simulink model "Observer_Controller"  (R2022a)
settings: Solver=ode45  StartTime=0.0  StopTime=20  RelTol=1e-3
values from neighbouring files (symbols this model uses):
  A = [0 0 1 0 0 ... (first row only)    [DesignProjectP2.m]    (also in DesignProjectP3.m; DesignProject_OffsetP3.m; mpc_example_regulation.m = [ 	 0,       0,              1,  0, 0; 	 0,       0,        ; mpc_example_tracking.m = [ 	 0,       0,              1,  0, 0; 	 0,       0,        )
  A_11 = A_measured(:,1:2)    [DesignProjectP2.m]
  A_12 = A_measured(:,3:5)    [DesignProjectP2.m]
  A_21 = A_estimated(:,1:2)    [DesignProjectP2.m]
  A_22 = A_estimated(:,3:5)    [DesignProjectP2.m]
  absolute_encoder_counts_per_revolution = 4096    [ELEN90064_Project_Parameters.m]
  B = [0;0;0;0;1/La]    [DesignProjectP2.m]    (also in DesignProjectP3.m; DesignProject_OffsetP3.m; mpc_example_regulation.m = [0; 0; 0; 0; 1/La]; mpc_example_tracking.m = [0; 0; 0; 0; 1/La])
  B_1 = [Dp.b(1); Dp.b(2)]    [DesignProjectP2.m]
  B_2 = [Dp.b(3); Dp.b(4); Dp.b(5)]    [DesignProjectP2.m]
  C = [1 0 0 0 0 ... (first row only)    [DesignProjectP2.m]    (also in DesignProjectP3.m; DesignProject_OffsetP3.m; mpc_example_regulation.m; mpc_example_tracking.m)
  init = [theta_m_init; theta_l_init; thetadot_m_init; thetadot_l_init; Ia_init]    [ELEN90064_Project_Parameters.m]
  J_r = place(A_22', A_12', obsz)'    [DesignProjectP2.m]
  K = K(2:6)    [DesignProjectP2.m]    (also in DesignProjectP3.m; DesignProject_OffsetP3.m = K_dist(2:6); phase2_emc.m = place(A,B,desired_poles))
  K_disc = K_disc(2:6)    [DesignProjectP2.m]    (also in DesignProject_OffsetP3.m = Kr_disc(2:6))
  Ki = K(1)    [DesignProjectP2.m]    (also in DesignProjectP3.m; DesignProject_OffsetP3.m = K_dist(1))
  Ki_disc = K_disc(1)    [DesignProjectP2.m]    (also in DesignProject_OffsetP3.m = Kr_disc(1))
  L = place(A', C', observer_poles)'    [DesignProjectP2.m]    (also in DesignProjectP3.m; DesignProject_OffsetP3.m = L_t'; phase2_emc.m = place(A',C',desired_obsv_poles)')
  theta_l_init = deg2rad(0)    [ELEN90064_Project_Parameters.m]    (also in mpc_example_regulation.m; mpc_example_tracking.m)
  vision_fps = 50    [ELEN90064_Project_Parameters.m]
settings Model: Creator=Admin  LastModifiedBy=Admin

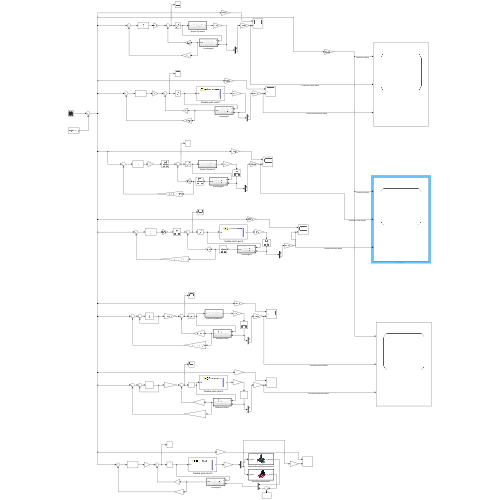
[thumbnail: Simulink's stored preview of the top-level diagram]
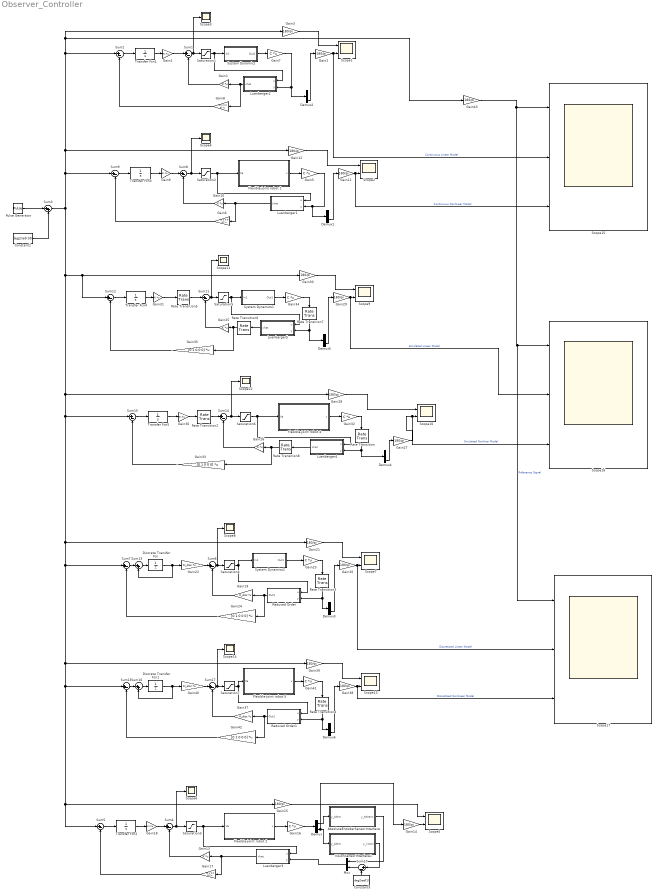
== system Observer_Controller ==
  AbsoluteEncoderSensorInterface : Subsystem  TreatAsAtomicUnit=on
      mask Display: image('$imagefile'); % Use "Edit Image" on toolstrip to change.
  Constant1 : Constant  Value=deg2rad(30)
  Constant3 : Constant  Value=deg2rad(1)
  Demux{,1..6} (7 alike) : Demux  Outputs=2
  Discrete Transfer Fcn : DiscreteTransferFcn  Denominator=[1 0]
  Discrete Transfer Fcn1 : DiscreteTransferFcn  Denominator=[1 0]
  Flexible-joint robot 1 : Subsystem
      mask Display: image('$imagefile'); % Use "Edit Image" on toolstrip to change.
  Flexible-joint robot 2 : Subsystem
      mask Display: image('$imagefile'); % Use "Edit Image" on toolstrip to change.
  Flexible-joint robot 4 : Subsystem
      mask Display: image('$imagefile'); % Use "Edit Image" on toolstrip to change.
  Flexible-joint robot 5 : Subsystem
      mask Display: image('$imagefile'); % Use "Edit Image" on toolstrip to change.
  Gain{1,10,13,25..26} (5 alike) : Gain  Gain=K  Multiplication=Matrix(K*u)
  Gain{2..3,11..12,14..15,20..21,27..30,38..39,43} (15 alike) : Gain  Gain=180/pi
  Gain{5,7,16,23,32,34,41} (7 alike) : Gain  Gain=C  Multiplication=Matrix(K*u)
  Gain{6,8,17,24,33,35,42} (7 alike) : Gain  Gain=[0 1 0 0 0]  Multiplication=Matrix(K*u)
  Gain{4,9,18,31,36} (5 alike) : Gain  Gain=Ki  Multiplication=Matrix(K*u)
  Gain19 : Gain  Gain=K_disc  Multiplication=Matrix(K*u)
  Gain22 : Gain  Gain=Ki_disc  Multiplication=Matrix(K*u)
  Gain37 : Gain  Gain=K_disc  Multiplication=Matrix(K*u)
  Gain40 : Gain  Gain=Ki_disc  Multiplication=Matrix(K*u)
  Luenberger1 : Subsystem  TreatAsAtomicUnit=on
  Luenberger2 : Subsystem  TreatAsAtomicUnit=on
  Luenberger3 : Subsystem  TreatAsAtomicUnit=on
  Luenberger4 : Subsystem  TreatAsAtomicUnit=on
  Luenberger5 : Subsystem  TreatAsAtomicUnit=on
  Mux : Mux  Inputs=2
  Pulse Generator : DiscretePulseGenerator  PulseType=Time based  Amplitude=deg2rad(30)  Period=5  PulseWidth=50
  Rate Transition{,2..8} (8 alike) : RateTransition  OutPortSampleTime=T
  Reduced Order : Subsystem  TreatAsAtomicUnit=on
  Reduced Order1 : Subsystem  TreatAsAtomicUnit=on
  Saturation{1..7} (7 alike) : Saturate  UpperLimit=6  LowerLimit=-6
  Scope{1..2,5,7,9..10,13} (7 alike) : Scope  NumInputPorts=2
  Scope{3..4,6,8,11..12,14} (7 alike) : Scope
  Scope15 : Scope  NumInputPorts=3
  Scope16 : Scope  NumInputPorts=3
  Scope17 : Scope  NumInputPorts=3
  Sum{1..2,4..12,14..15,17..18} (15 alike) : Sum  Inputs=|+-
  Sum13 : Sum  Inputs=|++
  Sum16 : Sum  Inputs=|++
  Sum3 : Sum  Inputs=|++
  System Dynamics : Subsystem  TreatAsAtomicUnit=on
  System Dynamics1 : Subsystem  TreatAsAtomicUnit=on
  System Dynamics2 : Subsystem  TreatAsAtomicUnit=on
  Transfer Fcn{1..5} (5 alike) : TransferFcn  Denominator=[1 0]
  VisionSensorInterface1 : Subsystem  TreatAsAtomicUnit=on
      mask Display: image('$imagefile'); % Use "Edit Image" on toolstrip to change.
  wires:
  Sum8/1 -> Scope4/1, Saturation2/1
  Saturation2/1 -> Luenberger1/1(u), Flexible-joint robot 1/1(Va)
  Sum9/1 -> Transfer Fcn3/1
  Gain10/1 -> Sum8/2
  Transfer Fcn3/1 -> Gain9/1
  Flexible-joint robot 1/1(x) -> Gain5/1
  Gain12/1 -> Scope2/1
  Gain11/1 -> Scope15/3, Scope2/2  "Continuous Nonlinear Model"
  Gain5/1 -> Demux1/1, Luenberger1/2(y)
  Luenberger1/1(xhat) -> Gain6/1, Gain10/1
  Gain6/1 -> Sum9/2
  Gain9/1 -> Sum8/1
  Gain2/1 -> Scope15/2, Scope1/2  "Continuous Linear Model"
  Gain3/1 -> Scope1/1
  Transfer Fcn1/1 -> Gain4/1
  Gain1/1 -> Sum1/2
  Sum2/1 -> Transfer Fcn1/1
  Sum1/1 -> Scope3/1, Saturation1/1
  Gain8/1 -> Sum2/2
  Gain4/1 -> Sum1/1
  Saturation1/1 -> Luenberger2/1(u), System Dynamics/1(In1)
  Luenberger2/1(xhat) -> Gain8/1, Gain1/1
  Pulse Generator/1 -> Sum3/1
  System Dynamics/1(Out1) -> Gain7/1
  Luenberger3/1(xhat) -> Gain17/1, Gain13/1
  Saturation3/1 -> Luenberger3/1(u), Flexible-joint robot 2/1(Va)
  Flexible-joint robot 2/1(x) -> Gain16/1
  Gain13/1 -> Sum4/2
  Gain14/1 -> Scope5/2
  Gain18/1 -> Sum4/1
  Sum5/1 -> Transfer Fcn2/1
  Sum4/1 -> Scope6/1, Saturation3/1
  Transfer Fcn2/1 -> Gain18/1
  Gain17/1 -> Sum5/2
  Gain15/1 -> Scope5/1
  Constant1/1 -> Sum3/2
  Gain16/1 -> Demux/1
  Demux/1 -> AbsoluteEncoderSensorInterface/1(y_plant)
  AbsoluteEncoderSensorInterface/1(y_absenc) -> Mux/1
  Demux/2 -> Gain14/1, VisionSensorInterface1/1(y_plant)
  Mux/1 -> Luenberger3/2(y)
  System Dynamics2/1(Out1) -> Gain23/1
  Reduced Order/1(Out1) -> Gain24/1, Gain19/1
  Saturation4/1 -> System Dynamics2/1(In1), Reduced Order/1(u)
  Gain22/1 -> Sum6/1
  Gain24/1 -> Sum7/2
  Sum6/1 -> Saturation4/1, Scope8/1
  Gain19/1 -> Sum6/2
  Gain21/1 -> Scope7/1
  Gain20/1 -> Scope17/2, Scope7/2  "Discretised Linear Model"
  VisionSensorInterface1/1(y_vision) -> Sum10/1
  Constant3/1 -> Sum10/2
  Sum10/1 -> Mux/2
  Demux1/2 -> Gain11/1
  Sum13/1 -> Discrete Transfer Fcn/1
  Discrete Transfer Fcn/1 -> Gain22/1, Sum13/2
  Sum7/1 -> Sum13/1
  Demux2/2 -> Gain2/1
  Gain7/1 -> Demux2/1, Luenberger2/2(y)
  Gain23/1 -> Rate Transition3/1
  Demux3/2 -> Gain20/1
  Gain34/1 -> Rate Transition7/1
  Demux5/2 -> Gain29/1
  Demux4/2 -> Gain27/1
  System Dynamics1/1(Out1) -> Gain34/1
  Luenberger5/1(xhat) -> Rate Transition6/1
  Saturation5/1 -> System Dynamics1/1(In1), Luenberger5/1(u)
  Gain31/1 -> Rate Transition5/1
  Gain35/1 -> Sum12/2
  Sum11/1 -> Saturation5/1, Scope11/1
  Sum12/1 -> Transfer Fcn4/1
  Gain25/1 -> Sum11/2
  Transfer Fcn4/1 -> Gain31/1
  Gain30/1 -> Scope9/1
  Gain29/1 -> Scope16/2, Scope9/2  "Emulated Linear Model"
  Gain36/1 -> Rate Transition2/1
  Gain33/1 -> Sum15/2
  Luenberger4/1(xhat) -> Rate Transition8/1
  Gain32/1 -> Rate Transition/1
  Gain27/1 -> Scope16/3, Scope10/2  "Emulated Nonliner Model"
  Gain28/1 -> Scope10/1
  Flexible-joint robot 4/1(x) -> Gain32/1
  Transfer Fcn5/1 -> Gain36/1
  Sum15/1 -> Transfer Fcn5/1
  Saturation6/1 -> Flexible-joint robot 4/1(Va), Luenberger4/1(u)
  Sum14/1 -> Saturation6/1, Scope12/1
  Rate Transition/1 -> Demux4/1, Luenberger4/2(y)
  Gain26/1 -> Sum14/2
  Rate Transition2/1 -> Sum14/1
  Sum3/1 -> Gain12/1, Gain3/1, Gain43/1, Sum2/1, Sum9/1, Sum12/1, Gain30/1, Gain28/1, Gain21/1, Gain39/1, Sum5/1, Gain15/1, Sum18/1, Sum7/1, Sum15/1
  Demux6/2 -> Gain38/1
  Gain41/1 -> Rate Transition4/1
  Sum18/1 -> Sum16/1
  Discrete Transfer Fcn1/1 -> Sum16/2, Gain40/1
  Sum16/1 -> Discrete Transfer Fcn1/1
  Gain38/1 -> Scope17/3, Scope13/2  "Discretised Nonlinear Model"
  Gain39/1 -> Scope13/1
  Gain37/1 -> Sum17/2
  Sum17/1 -> Scope14/1, Saturation7/1
  Gain42/1 -> Sum18/2
  Gain40/1 -> Sum17/1
  Saturation7/1 -> Reduced Order1/1(u), Flexible-joint robot 5/1(Va)
  Reduced Order1/1(Out1) -> Gain37/1, Gain42/1
  Flexible-joint robot 5/1(x) -> Gain41/1
  Rate Transition3/1 -> Demux3/1, Reduced Order/2(y)
  Rate Transition4/1 -> Demux6/1, Reduced Order1/2(y)
  Rate Transition5/1 -> Sum11/1
  Rate Transition6/1 -> Gain35/1, Gain25/1
  Rate Transition7/1 -> Luenberger5/2(y), Demux5/1
  Gain43/1 -> Scope17/1, Scope16/1, Scope15/1  "Reference Signal"
  Rate Transition8/1 -> Gain33/1, Gain26/1

== system Observer_Controller/AbsoluteEncoderSensorInterface ==
  note: Notes:
      | > This sensor block is protected.
      | > The AbsoluteEncoderSensor.slxp file needs to be on the Matlab path in order to simulate this sensor.
      | > You should have download the .slpx file appropriate for you operating system {Windows, Mac, Linux}.
      | > The constant parameters on the left are set in the " ELEN90064_Project_Parameters.m " script.
      | > The sensors appendix in project description provides a 1-page summary of the sensor model and of how each parameters relates to the expected performance of the sensor.
      | > You should read the relevant page of that appendix before using this sensor.
  y_plant : Inport
  AbsoluteEncoderSensor : ModelReference  ModelNameDialog=AbsoluteEncoderSensor.slxp  ModelReferenceVersion=1.16  CopyOfModelProtected=on
  NUMBER OF COUNTS PER REVOLUTION : Constant  Value=absolute_encoder_counts_per_revolution
  y_absenc : Outport
  wires:
  NUMBER OF COUNTS PER REVOLUTION/1 -> AbsoluteEncoderSensor/1
  y_plant/1 -> AbsoluteEncoderSensor/2
  AbsoluteEncoderSensor/1 -> y_absenc/1

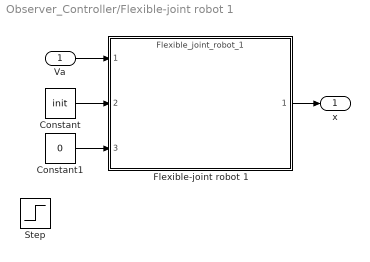
== system Observer_Controller/Flexible-joint robot 1 ==
  Va : Inport
  Constant : Constant  Value=init
  Constant1 : Constant  Value=0
  Flexible-joint robot 1 : ModelReference  ModelNameDialog=Flexible_joint_robot_1  ModelReferenceVersion=1.65  CopyOfModelProtected=on
  Step : Step  After=0.05  SampleTime=0
  x : Outport
  wires:
  Constant/1 -> Flexible-joint robot 1/2
  Constant1/1 -> Flexible-joint robot 1/3
  Flexible-joint robot 1/1 -> x/1
  Va/1 -> Flexible-joint robot 1/1

== system Observer_Controller/Flexible-joint robot 2 ==
  Va : Inport
  Constant : Constant  Value=init
  Constant1 : Constant  Value=0
  Flexible-joint robot 1 : ModelReference  ModelNameDialog=Flexible_joint_robot_1  ModelReferenceVersion=1.65  CopyOfModelProtected=on
  x : Outport
  wires:
  Constant/1 -> Flexible-joint robot 1/2
  Constant1/1 -> Flexible-joint robot 1/3
  Flexible-joint robot 1/1 -> x/1
  Va/1 -> Flexible-joint robot 1/1

== system Observer_Controller/Flexible-joint robot 4 ==
  Va : Inport
  Constant : Constant  Value=init
  Constant1 : Constant  Value=0
  Flexible-joint robot 1 : ModelReference  ModelNameDialog=Flexible_joint_robot_1  ModelReferenceVersion=1.65  CopyOfModelProtected=on
  Step : Step  After=0.05  SampleTime=0
  x : Outport
  wires:
  Va/1 -> Flexible-joint robot 1/1
  Flexible-joint robot 1/1 -> x/1
  Constant1/1 -> Flexible-joint robot 1/3
  Constant/1 -> Flexible-joint robot 1/2

== system Observer_Controller/Flexible-joint robot 5 ==
  Va : Inport
  Constant : Constant  Value=init
  Constant1 : Constant  Value=0
  Flexible-joint robot 1 : ModelReference  ModelNameDialog=Flexible_joint_robot_1  ModelReferenceVersion=1.65  CopyOfModelProtected=on
  Step : Step  After=0.05  SampleTime=0
  x : Outport
  wires:
  Constant/1 -> Flexible-joint robot 1/2
  Constant1/1 -> Flexible-joint robot 1/3
  Flexible-joint robot 1/1 -> x/1
  Va/1 -> Flexible-joint robot 1/1

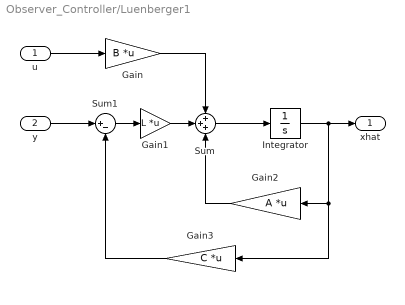
== system Observer_Controller/Luenberger1 ==
  u : Inport
  y : Inport  Port=2
  Gain : Gain  Gain=B  Multiplication=Matrix(K*u) (u vector)
  Gain1 : Gain  Gain=L  Multiplication=Matrix(K*u) (u vector)
  Gain2 : Gain  Gain=A  Multiplication=Matrix(K*u) (u vector)
  Gain3 : Gain  Gain=C  Multiplication=Matrix(K*u) (u vector)
  Integrator : Integrator
  Sum : Sum  Inputs=+++
  Sum1 : Sum  Inputs=|+-
  xhat : Outport
  wires:
  u/1 -> Gain/1
  Gain/1 -> Sum/1
  y/1 -> Sum1/1
  Sum1/1 -> Gain1/1
  Gain1/1 -> Sum/2
  Sum/1 -> Integrator/1
  Integrator/1 -> Gain3/1, Gain2/1, xhat/1
  Gain2/1 -> Sum/3
  Gain3/1 -> Sum1/2

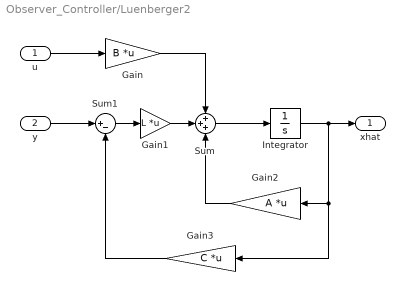
== system Observer_Controller/Luenberger2 ==
  u : Inport
  y : Inport  Port=2
  Gain : Gain  Gain=B  Multiplication=Matrix(K*u) (u vector)
  Gain1 : Gain  Gain=L  Multiplication=Matrix(K*u) (u vector)
  Gain2 : Gain  Gain=A  Multiplication=Matrix(K*u) (u vector)
  Gain3 : Gain  Gain=C  Multiplication=Matrix(K*u) (u vector)
  Integrator : Integrator
  Sum : Sum  Inputs=+++
  Sum1 : Sum  Inputs=|+-
  xhat : Outport
  wires:
  u/1 -> Gain/1
  Gain/1 -> Sum/1
  y/1 -> Sum1/1
  Sum1/1 -> Gain1/1
  Gain1/1 -> Sum/2
  Sum/1 -> Integrator/1
  Integrator/1 -> Gain3/1, Gain2/1, xhat/1
  Gain2/1 -> Sum/3
  Gain3/1 -> Sum1/2

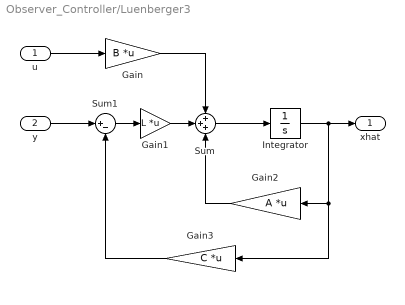
== system Observer_Controller/Luenberger3 ==
  u : Inport
  y : Inport  Port=2
  Gain : Gain  Gain=B  Multiplication=Matrix(K*u) (u vector)
  Gain1 : Gain  Gain=L  Multiplication=Matrix(K*u) (u vector)
  Gain2 : Gain  Gain=A  Multiplication=Matrix(K*u) (u vector)
  Gain3 : Gain  Gain=C  Multiplication=Matrix(K*u) (u vector)
  Integrator : Integrator
  Sum : Sum  Inputs=+++
  Sum1 : Sum  Inputs=|+-
  xhat : Outport
  wires:
  u/1 -> Gain/1
  Gain/1 -> Sum/1
  y/1 -> Sum1/1
  Sum1/1 -> Gain1/1
  Gain1/1 -> Sum/2
  Sum/1 -> Integrator/1
  Integrator/1 -> Gain3/1, Gain2/1, xhat/1
  Gain2/1 -> Sum/3
  Gain3/1 -> Sum1/2

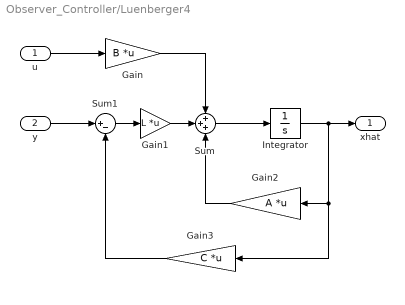
== system Observer_Controller/Luenberger4 ==
  u : Inport
  y : Inport  Port=2
  Gain : Gain  Gain=B  Multiplication=Matrix(K*u) (u vector)
  Gain1 : Gain  Gain=L  Multiplication=Matrix(K*u) (u vector)
  Gain2 : Gain  Gain=A  Multiplication=Matrix(K*u) (u vector)
  Gain3 : Gain  Gain=C  Multiplication=Matrix(K*u) (u vector)
  Integrator : Integrator
  Sum : Sum  Inputs=+++
  Sum1 : Sum  Inputs=|+-
  xhat : Outport
  wires:
  Gain3/1 -> Sum1/2
  Gain2/1 -> Sum/3
  Integrator/1 -> xhat/1, Gain2/1, Gain3/1
  Sum/1 -> Integrator/1
  Gain1/1 -> Sum/2
  Sum1/1 -> Gain1/1
  y/1 -> Sum1/1
  Gain/1 -> Sum/1
  u/1 -> Gain/1

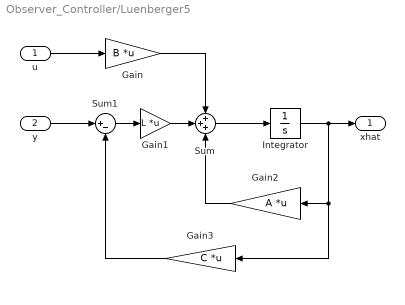
== system Observer_Controller/Luenberger5 ==
  u : Inport
  y : Inport  Port=2
  Gain : Gain  Gain=B  Multiplication=Matrix(K*u) (u vector)
  Gain1 : Gain  Gain=L  Multiplication=Matrix(K*u) (u vector)
  Gain2 : Gain  Gain=A  Multiplication=Matrix(K*u) (u vector)
  Gain3 : Gain  Gain=C  Multiplication=Matrix(K*u) (u vector)
  Integrator : Integrator
  Sum : Sum  Inputs=+++
  Sum1 : Sum  Inputs=|+-
  xhat : Outport
  wires:
  Gain3/1 -> Sum1/2
  Gain2/1 -> Sum/3
  Integrator/1 -> xhat/1, Gain2/1, Gain3/1
  Sum/1 -> Integrator/1
  Gain1/1 -> Sum/2
  Sum1/1 -> Gain1/1
  y/1 -> Sum1/1
  Gain/1 -> Sum/1
  u/1 -> Gain/1

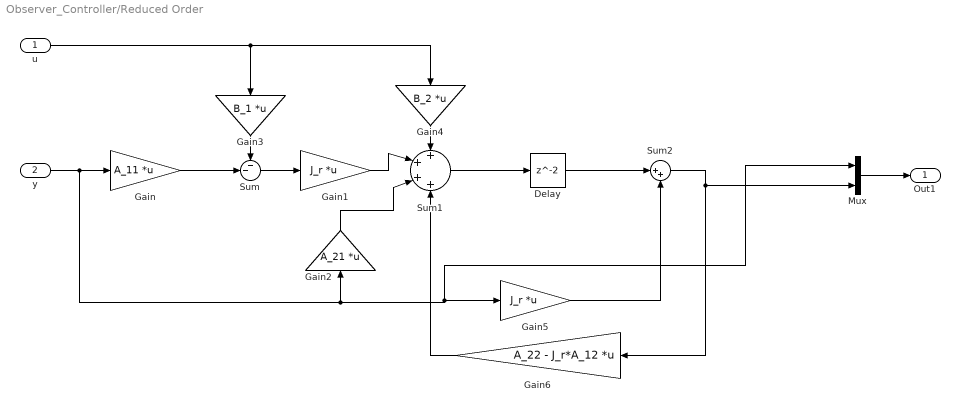
== system Observer_Controller/Reduced Order ==
  u : Inport
  y : Inport  Port=2
  Delay : Delay
  Gain : Gain  Gain=A_11  Multiplication=Matrix(K*u) (u vector)
  Gain1 : Gain  Gain=J_r  Multiplication=Matrix(K*u) (u vector)
  Gain2 : Gain  Gain=A_21  Multiplication=Matrix(K*u) (u vector)
  Gain3 : Gain  Gain=B_1  Multiplication=Matrix(K*u) (u vector)
  Gain4 : Gain  Gain=B_2  Multiplication=Matrix(K*u) (u vector)
  Gain5 : Gain  Gain=J_r  Multiplication=Matrix(K*u) (u vector)
  Gain6 : Gain  Gain=A_22 - J_r*A_12  Multiplication=Matrix(K*u) (u vector)
  Mux : Mux  Inputs=2
  Sum : Sum  Inputs=--|
  Sum1 : Sum  Inputs=++++
  Sum2 : Sum  Inputs=|++
  Out1 : Outport
  wires:
  u/1 -> Gain4/1, Gain3/1
  y/1 -> Gain2/1, Mux/1, Gain5/1, Gain/1
  Gain/1 -> Sum/2
  Sum/1 -> Gain1/1
  Gain1/1 -> Sum1/2
  Gain2/1 -> Sum1/3
  Gain3/1 -> Sum/1
  Gain4/1 -> Sum1/1
  Sum1/1 -> Delay/1
  Gain5/1 -> Sum2/2
  Delay/1 -> Sum2/1
  Gain6/1 -> Sum1/4
  Sum2/1 -> Gain6/1, Mux/2
  Mux/1 -> Out1/1

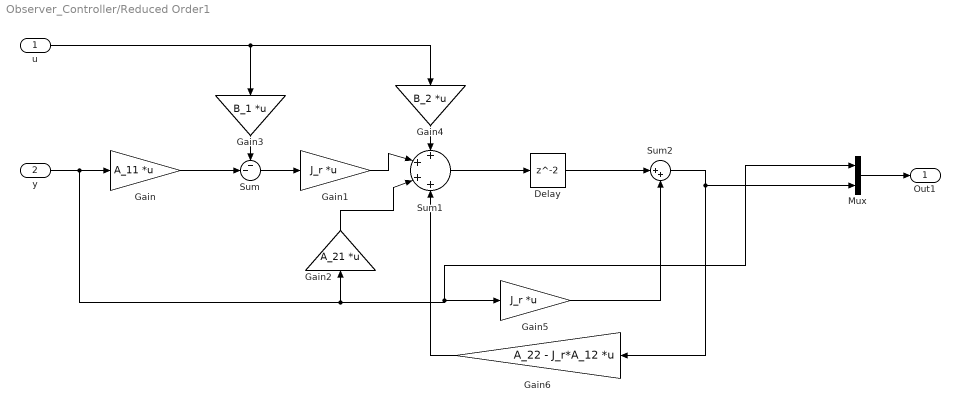
== system Observer_Controller/Reduced Order1 ==
  u : Inport
  y : Inport  Port=2
  Delay : Delay
  Gain : Gain  Gain=A_11  Multiplication=Matrix(K*u) (u vector)
  Gain1 : Gain  Gain=J_r  Multiplication=Matrix(K*u) (u vector)
  Gain2 : Gain  Gain=A_21  Multiplication=Matrix(K*u) (u vector)
  Gain3 : Gain  Gain=B_1  Multiplication=Matrix(K*u) (u vector)
  Gain4 : Gain  Gain=B_2  Multiplication=Matrix(K*u) (u vector)
  Gain5 : Gain  Gain=J_r  Multiplication=Matrix(K*u) (u vector)
  Gain6 : Gain  Gain=A_22 - J_r*A_12  Multiplication=Matrix(K*u) (u vector)
  Mux : Mux  Inputs=2
  Sum : Sum  Inputs=--|
  Sum1 : Sum  Inputs=++++
  Sum2 : Sum  Inputs=|++
  Out1 : Outport
  wires:
  Mux/1 -> Out1/1
  Sum2/1 -> Mux/2, Gain6/1
  Gain6/1 -> Sum1/4
  Delay/1 -> Sum2/1
  Gain5/1 -> Sum2/2
  Sum1/1 -> Delay/1
  Gain4/1 -> Sum1/1
  Gain3/1 -> Sum/1
  Gain2/1 -> Sum1/3
  Gain1/1 -> Sum1/2
  Sum/1 -> Gain1/1
  Gain/1 -> Sum/2
  y/1 -> Gain/1, Gain5/1, Mux/1, Gain2/1
  u/1 -> Gain3/1, Gain4/1

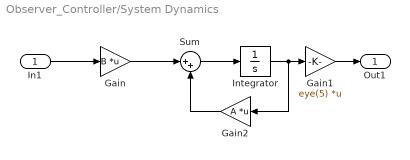
== system Observer_Controller/System Dynamics ==
  In1 : Inport
  Gain : Gain  Gain=B  Multiplication=Matrix(K*u)
  Gain1 : Gain  Gain=eye(5)  Multiplication=Matrix(K*u)
  Gain2 : Gain  Gain=A  Multiplication=Matrix(K*u)
  Integrator : Integrator
  Sum : Sum  Inputs=|++
  Out1 : Outport
  wires:
  In1/1 -> Gain/1
  Gain/1 -> Sum/1
  Sum/1 -> Integrator/1
  Integrator/1 -> Gain2/1, Gain1/1
  Gain1/1 -> Out1/1
  Gain2/1 -> Sum/2

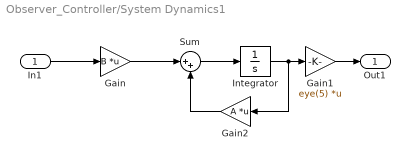
== system Observer_Controller/System Dynamics1 ==
  In1 : Inport
  Gain : Gain  Gain=B  Multiplication=Matrix(K*u)
  Gain1 : Gain  Gain=eye(5)  Multiplication=Matrix(K*u)
  Gain2 : Gain  Gain=A  Multiplication=Matrix(K*u)
  Integrator : Integrator
  Sum : Sum  Inputs=|++
  Out1 : Outport
  wires:
  Gain2/1 -> Sum/2
  Gain1/1 -> Out1/1
  Integrator/1 -> Gain1/1, Gain2/1
  Sum/1 -> Integrator/1
  Gain/1 -> Sum/1
  In1/1 -> Gain/1

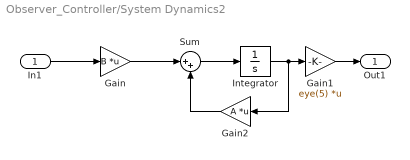
== system Observer_Controller/System Dynamics2 ==
  In1 : Inport
  Gain : Gain  Gain=B  Multiplication=Matrix(K*u)
  Gain1 : Gain  Gain=eye(5)  Multiplication=Matrix(K*u)
  Gain2 : Gain  Gain=A  Multiplication=Matrix(K*u)
  Integrator : Integrator
  Sum : Sum  Inputs=|++
  Out1 : Outport
  wires:
  In1/1 -> Gain/1
  Gain/1 -> Sum/1
  Sum/1 -> Integrator/1
  Integrator/1 -> Gain2/1, Gain1/1
  Gain1/1 -> Out1/1
  Gain2/1 -> Sum/2

== system Observer_Controller/VisionSensorInterface1 ==
  note: Notes:
      | > This sensor block is protected.
      | > The VisionSensor.slxp file needs to be on the Matlab path in order to simulate this sensor.
      | > You should have download the .slpx file appropriate for you operating system {Windows, Mac, Linux}.
      | > The constant parameters on the left are set in the "ELEN90064_Project_Parameters.m" script.
      | > The sensors appendix in project description provides a 1-page summary of the sensor model and of how each parameters relates to the expected performance of the sensor.
      | > You should read the relevant page of that appendix before using this sensor.
  y_plant : Inport
  INITIAL LINK ANGLE [rad] : Constant  Value=theta_l_init
  VISION FRAME RATE [fps] : Constant  Value=vision_fps
  VisionSensor : ModelReference  ModelNameDialog=VisionSensor.slxp  ModelReferenceVersion=1.19  CopyOfModelProtected=on
  y_vision : Outport
  wires:
  VisionSensor/1 -> y_vision/1
  y_plant/1 -> VisionSensor/3
  INITIAL LINK ANGLE [rad]/1 -> VisionSensor/2
  VISION FRAME RATE [fps]/1 -> VisionSensor/1
